simulink model "Sim_Helikopter"  (R2015b)
settings: Solver=ode113  StartTime=0.0  StopTime=50  RelTol=1e-2
PostLoadFcn:
  | , if any(exist('dsrtsu_mdlpostloadfcn', 'file') == [2, 3, 6]), try dsrtsu_mdlpostloadfcn('Execute', bdroot); catch fprintf('Error in PostLoadFcn (dsrtsu_mdlpostloadfcn) for model "%s":\n %s\n', bdroot, lasterr); end, end,
InitFcn:
  | Initialisierung
values from neighbouring files (symbols this model uses):
  initCond = block.DialogPrm(2).Data    [ROFLcopter_modell_S.m]    (also in set_parameter_vollstaendigesModell.m = [0,0,q20,0,0,0,0,0,0,0,0,0]')
  parameters = p    [set_parameter_vollstaendigesModell.m]
  q10e = 0    [Initialisierung.m]
  q1d = 2*pi    (= 6.28318530718)    [Initialisierung.m]
  q20e = 0.319187912478128    (= 0.319187912478)    [Initialisierung.m]
  q2d = 0    [Initialisierung.m]
  sysPar = block.DialogPrm(1).Data    [ROFLcopter_modell_S.m]
  Ta = 1e-3    (= 0.001)    [Initialisierung.m]    (also in Initialisierung_bitte_vervollstaendigen.m)
undefined symbols (not defined in the file or in its folder): F2U, Fout, regPar
settings Model: DSRTSU_INTERNAL_RTI_VER=340  DSRTSU_INTERNAL_RTI_TYPE=rti1103  ExtModeArmWhenConnect=off  Creator=tk  LastModifiedBy=Andreas
settings DataIOCC: SaveFormat=Array  SignalLoggingSaveFormat=ModelDataLogs  SignalLoggingName=sigsOut
settings OptimizationCC: ConditionallyExecuteInputs=off  OptimizeBlockIOStorage=off  BufferReuse=off  GlobalBufferReuse=off  ExpressionFolding=off  ExpressionDepthLimit=2147483647  LocalBlockOutputs=off  InitFltsAndDblsToZero=on
settings DebuggingCC: SaveWithParameterizedLinksMsg=none  UnderspecifiedInitializationDetection=Classic  MergeDetectMultiDrivingBlocksExec=none  SignalResolutionControl=TryResolveAllWithWarning  MultiTaskDSMMsg=warning  MultiTaskCondExecSysMsg=none  FcnCallInpInsideContextMsg=UseLocalSettings  StateNameClashWarn=warning
settings HardwareCC: ProdBitPerPointer=32  ProdLargestAtomicFloat=None  ProdIntDivRoundTo=Undefined  ProdEndianess=Unspecified  ProdWordSize=32  ProdHWDeviceType=32-bit Generic  TargetBitPerLong=64  TargetBitPerPointer=64  TargetLongLongMode=on  TargetIntDivRoundTo=Zero  TargetEndianess=LittleEndian  TargetWordSize=64  TargetHWDeviceType=MATLAB Host  ProdEqTarget=off
settings SFSimCC: SimParseCustomCode=off
settings RTWCC: SystemTargetFile=rtwsfcn.tlc  TemplateMakefile=rtwsfcn_default_tmf  Description=S-function Target  RetainRTWFile=on  RTWCompilerOptimization=on
settings STFCustomTargetCC: ModelReferenceCompliant=off  CompOptLevelCompliant=on  ConcurrentExecutionCompliant=off  MATLABClassNameForMDSCustomization=Simulink.SoftwareTarget.TargetSpecificTriggerConfigurationBase  CPPClassGenCompliant=off  SystemTargetFile=rtwsfcn.tlc
settings ConfigComp: CovModelRefEnable=Off

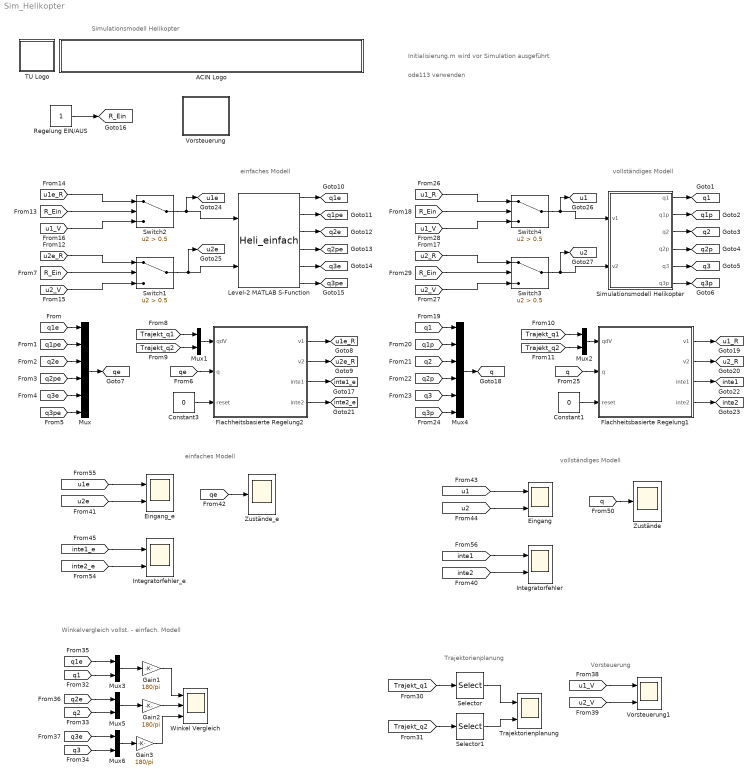
== system Sim_Helikopter ==
  note: ode113 verwenden
  note: Initialisierung.m wird vor Simulation ausgeführt
  note: vollständiges Modell
  note: einfaches Modell
  note: Simulationsmodell Helikopter
  note: Winkelvergleich vollst. - einfach. Modell
  note: Trajektorienplanung
  note: Vorsteuerung
  note: einfaches Modell
  note: vollständiges Modell
  ACIN Logo : Subsystem
      mask init:
      | s = get_param(gcb,'UserData');
      mask Display:
      | image(s.logo,[0 0 439 45]);
      | %axis image
  Constant1 : Constant  Value=0
  Constant3 : Constant  Value=0
  Eingang : Scope  NumInputPorts=2
  Eingang_e : Scope  NumInputPorts=2
  Flachheitsbasierte Regelung1 : MATLAB Function  TreatAsAtomicUnit=on
  Flachheitsbasierte Regelung2 : MATLAB Function  TreatAsAtomicUnit=on
  Gain1 : Gain  Gain=180/pi  SaturateOnIntegerOverflow=on  OutDataTypeStr=Inherit: Same as input  ParamDataTypeStr=Inherit: Same as input
  Gain2 : Gain  Gain=180/pi  SaturateOnIntegerOverflow=on  OutDataTypeStr=Inherit: Same as input  ParamDataTypeStr=Inherit: Same as input
  Gain3 : Gain  Gain=180/pi  SaturateOnIntegerOverflow=on  OutDataTypeStr=Inherit: Same as input  ParamDataTypeStr=Inherit: Same as input
  Integratorfehler : Scope  NumInputPorts=2
  Integratorfehler_e : Scope  NumInputPorts=2
  Level-2 MATLAB S-Function : M-S-Function  FunctionName=Heli_einfach  Parameters=sysPar.xR [sysPar.a1 sysPar.a2 sysPar.a3 sysPar.b1 sysPar.b2 sysPar.b3]
  Mux : Mux  Inputs=6
  Mux{1..3,5..6} (5 alike) : Mux  Inputs=2
  Mux4 : Mux  Inputs=6
  Regelung EIN/AUS : Constant
  Selector : Selector  InputPortWidth=5  IndexOptions=Index vector (dialog)  Indices=1  OutputSizes=1
  Selector1 : Selector  InputPortWidth=5  IndexOptions=Index vector (dialog)  Indices=1  OutputSizes=1
  Simulationsmodell Helikopter : Subsystem
  Switch{1..4} (4 alike) : Switch  Criteria=u2 > Threshold  Threshold=0.5
  TU Logo : Subsystem
      mask init:
      | s = get_param(gcb,'UserData');
      mask Display: image(s.logo,[0 0 45 45]);
  Trajektorienplanung : Scope  NumInputPorts=2
  Vorsteuerung : Subsystem
  Vorsteuerung1 : Scope  NumInputPorts=2
  Winkel Vergleich : Scope  NumInputPorts=3
  "Zustände " : Scope
  Zustände_e : Scope
  tag scope: R_Ein=global, inte1=global, inte1_e=global, inte2=global, inte2_e=global, q1=global, q1e=global, q1p=global, q1pe=global, q2=global, q2e=global, q2p=global, q2pe=global, q3=global, q3e=global, q3p=global, q3pe=global, q=global, qe=global, u1=global, u1_R=global, u1e=global, u1e_R=global, u2=global, u2_R=global, u2e=global, u2e_R=global
  wires:
  Simulationsmodell Helikopter/1(q1) -> [q1]
  Simulationsmodell Helikopter/2(q1p) -> [q1p]
  Simulationsmodell Helikopter/3(q2) -> [q2]
  Simulationsmodell Helikopter/4(q2p) -> [q2p]
  Simulationsmodell Helikopter/5(q3) -> [q3]
  Simulationsmodell Helikopter/6(q3p) -> [q3p]
  Mux/1 -> [qe]
  [q1e] -> Mux/1
  [q1pe] -> Mux/2
  [q2e] -> Mux/3
  [q2pe] -> Mux/4
  [q3e] -> Mux/5
  [q3pe] -> Mux/6
  Level-2 MATLAB S-Function/6 -> [q3pe]
  Level-2 MATLAB S-Function/5 -> [q3e]
  Level-2 MATLAB S-Function/4 -> [q2pe]
  Level-2 MATLAB S-Function/3 -> [q2e]
  Level-2 MATLAB S-Function/2 -> [q1pe]
  Level-2 MATLAB S-Function/1 -> [q1e]
  Mux4/1 -> [q]
  [q1] -> Mux4/1
  [q1p] -> Mux4/2
  [q2] -> Mux4/3
  [q2p] -> Mux4/4
  [q3] -> Mux4/5
  [q3p] -> Mux4/6
  Flachheitsbasierte Regelung1/1(v1) -> [u1_R]
  Flachheitsbasierte Regelung1/2(v2) -> [u2_R]
  Constant1/1 -> Flachheitsbasierte Regelung1/3(reset)
  [q] -> Flachheitsbasierte Regelung1/2(q)
  Flachheitsbasierte Regelung1/3(inte1) -> [inte1]
  Flachheitsbasierte Regelung1/4(inte2) -> [inte2]
  Flachheitsbasierte Regelung2/1(v1) -> [u1e_R]
  Flachheitsbasierte Regelung2/2(v2) -> [u2e_R]
  Constant3/1 -> Flachheitsbasierte Regelung2/3(reset)
  Mux1/1 -> Flachheitsbasierte Regelung2/1(qdV)
  [qe] -> Flachheitsbasierte Regelung2/2(q)
  Flachheitsbasierte Regelung2/3(inte1) -> [inte1_e]
  Flachheitsbasierte Regelung2/4(inte2) -> [inte2_e]
  Switch2/1 -> [u1e], Level-2 MATLAB S-Function/1
  [Trajekt_q1] -> Mux1/1
  [Trajekt_q2] -> Mux1/2
  [Trajekt_q1] -> Mux2/1
  [Trajekt_q2] -> Mux2/2
  Mux2/1 -> Flachheitsbasierte Regelung1/1(qdV)
  [R_Ein] -> Switch2/2
  [u1e_R] -> Switch2/1
  [u1_V] -> Switch2/3
  [R_Ein] -> Switch1/2
  [u2e_R] -> Switch1/1
  [u2_V] -> Switch1/3
  Switch1/1 -> [u2e], Level-2 MATLAB S-Function/2
  Switch4/1 -> [u1], Simulationsmodell Helikopter/1(v1)
  [R_Ein] -> Switch4/2
  [u1_R] -> Switch4/1
  [u1_V] -> Switch4/3
  [R_Ein] -> Switch3/2
  [u2_R] -> Switch3/1
  [u2_V] -> Switch3/3
  Switch3/1 -> [u2], Simulationsmodell Helikopter/2(v2)
  Regelung EIN/AUS/1 -> [R_Ein]
  [q3] -> Mux6/2
  [q2] -> Mux5/2
  [q1] -> Mux3/2
  [q3e] -> Mux6/1
  [q2e] -> Mux5/1
  [q1e] -> Mux3/1
  [u1_V] -> Vorsteuerung1/1
  [u2_V] -> Vorsteuerung1/2
  [u1] -> Eingang/1
  [u2] -> Eingang/2
  Gain1/1 -> Winkel Vergleich/1
  Mux3/1 -> Gain1/1
  Gain2/1 -> Winkel Vergleich/2
  Mux5/1 -> Gain2/1
  Mux6/1 -> Gain3/1
  Gain3/1 -> Winkel Vergleich/3
  [inte1] -> Integratorfehler/1
  [inte2] -> Integratorfehler/2
  [u1e] -> Eingang_e/1
  [u2e] -> Eingang_e/2
  [inte1_e] -> Integratorfehler_e/1
  [inte2_e] -> Integratorfehler_e/2
  [q] -> "Zustände "/1
  [qe] -> Zustände_e/1
  [Trajekt_q1] -> Selector/1
  Selector/1 -> Trajektorienplanung/1
  [Trajekt_q2] -> Selector1/1
  Selector1/1 -> Trajektorienplanung/2

== system Sim_Helikopter/ACIN Logo ==

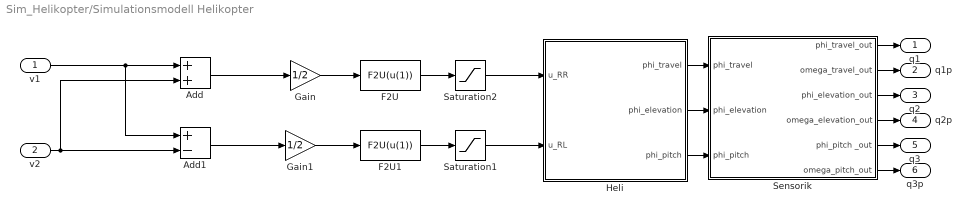
== system Sim_Helikopter/Simulationsmodell Helikopter ==
  v1 : Inport
  v2 : Inport  Port=2
  Add : Sum
  Add1 : Sum  Inputs=+-
  F2U : MATLABFcn  MATLABFcn=F2U(u(1))  OutputDimensions=1  Output1D=off
  F2U1 : MATLABFcn  MATLABFcn=F2U(u(1))  OutputDimensions=1  Output1D=off
  Gain : Gain  Gain=1/2
  Gain1 : Gain  Gain=1/2
  Heli : Subsystem
  Saturation1 : Saturate  UpperLimit=15  LowerLimit=-15
  Saturation2 : Saturate  UpperLimit=15  LowerLimit=-15
  Sensorik : Subsystem
  q1 : Outport
  q1p : Outport  Port=2
  q2 : Outport  Port=3
  q2p : Outport  Port=4
  q3 : Outport  Port=5
  q3p : Outport  Port=6
  wires:
  Saturation1/1 -> Heli/2(u_RL)
  Saturation2/1 -> Heli/1(u_RR)
  Heli/1(phi_travel) -> Sensorik/1(phi_travel)
  Heli/2(phi_elevation) -> Sensorik/2(phi_elevation)
  Heli/3(phi_pitch) -> Sensorik/3(phi_pitch)
  Sensorik/1(phi_travel_out) -> q1/1
  Sensorik/2(omega_travel_out) -> q1p/1
  Sensorik/3(phi_elevation_out) -> q2/1
  Sensorik/4(omega_elevation_out) -> q2p/1
  Sensorik/5(phi_pitch _out) -> q3/1
  Sensorik/6(omega_pitch_out) -> q3p/1
  v1/1 -> Add/1, Add1/1
  v2/1 -> Add/2, Add1/2
  Add/1 -> Gain/1
  Add1/1 -> Gain1/1
  Gain/1 -> F2U/1
  Gain1/1 -> F2U1/1
  F2U/1 -> Saturation2/1
  F2U1/1 -> Saturation1/1

== system Sim_Helikopter/TU Logo ==

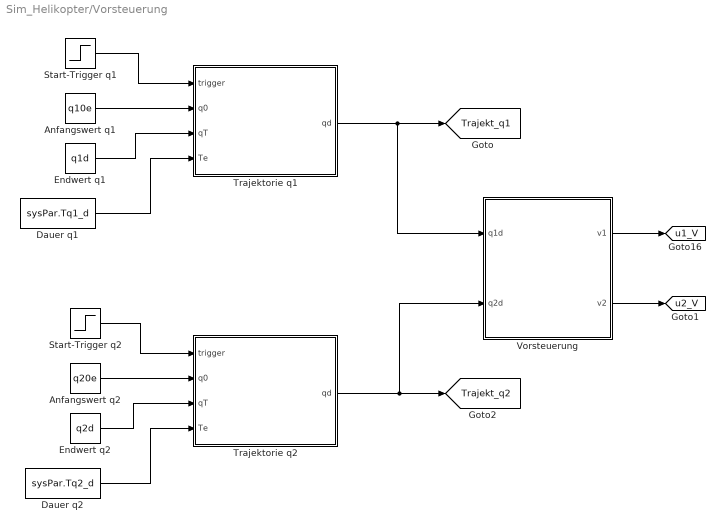
== system Sim_Helikopter/Vorsteuerung ==
  Anfangswert q1 : Constant  Value=q10e
  Anfangswert q2 : Constant  Value=q20e
  Dauer q1 : Constant  Value=sysPar.Tq1_d
  Dauer q2 : Constant  Value=sysPar.Tq2_d
  Endwert q1 : Constant  Value=q1d
  Endwert q2 : Constant  Value=q2d
  Start-Trigger q1 : Step  Time=sysPar.Tq1_s  SampleTime=0
  Start-Trigger q2 : Step  Time=sysPar.Tq2_s  SampleTime=0
  Trajektorie q1 : MATLAB Function  TreatAsAtomicUnit=on
  Trajektorie q2 : MATLAB Function  TreatAsAtomicUnit=on
  "Vorsteuerung " : MATLAB Function  TreatAsAtomicUnit=on
  tag scope: Trajekt_q1=global, Trajekt_q2=global, u1_V=global, u2_V=global
  wires:
  Start-Trigger q1/1 -> Trajektorie q1/1(trigger)
  Anfangswert q1/1 -> Trajektorie q1/2(q0)
  Endwert q1/1 -> Trajektorie q1/3(qT)
  Start-Trigger q2/1 -> Trajektorie q2/1(trigger)
  Anfangswert q2/1 -> Trajektorie q2/2(q0)
  Endwert q2/1 -> Trajektorie q2/3(qT)
  Trajektorie q1/1(qd) -> [Trajekt_q1], "Vorsteuerung "/1(q1d)
  Dauer q2/1 -> Trajektorie q2/4(Te)
  Dauer q1/1 -> Trajektorie q1/4(Te)
  Trajektorie q2/1(qd) -> [Trajekt_q2], "Vorsteuerung "/2(q2d)
  "Vorsteuerung "/2(v2) -> [u2_V]
  "Vorsteuerung "/1(v1) -> [u1_V]

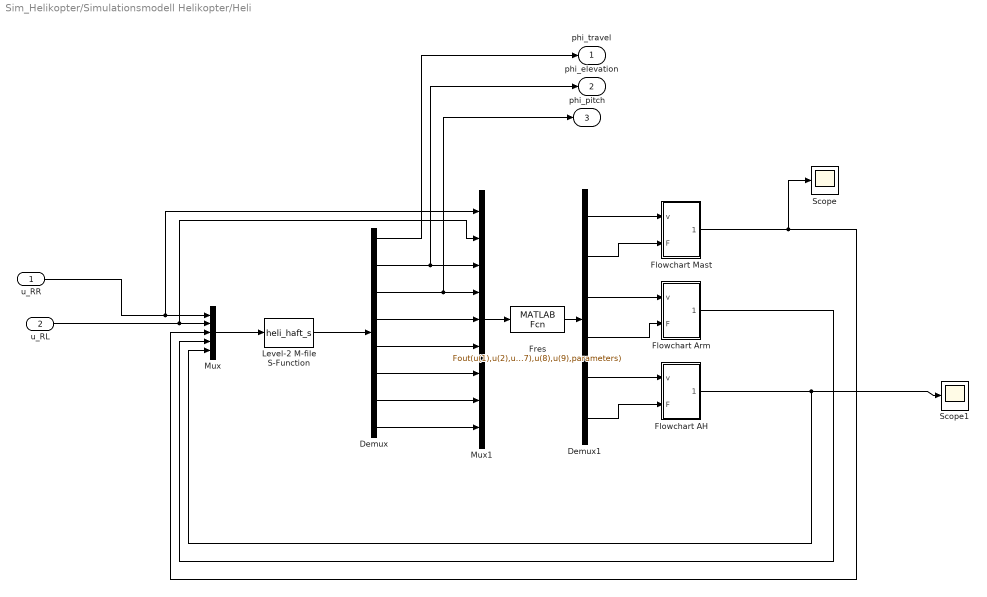
== system Sim_Helikopter/Simulationsmodell Helikopter/Heli ==
  u_RR : Inport
  u_RL : Inport  Port=2
  Demux : Demux  Outputs=8
  Demux1 : Demux  Outputs=6
  Flowchart AH : Subsystem
  Flowchart Arm : Subsystem
  Flowchart Mast : Subsystem
  Fres : MATLABFcn  MATLABFcn=Fout(u(1),u(2),u(3),u(4),u(5),u(6),u(7),u(8),u(9),parameters)  OutputDimensions=6  Output1D=off
  Level-2 M-file S-Function : M-S-Function  FunctionName=heli_haft_s  Parameters=initCond, parameters
  Mux : Mux  Inputs=5
  Mux1 : Mux  Inputs=9
  Scope : Scope
  Scope1 : Scope
  phi_travel : Outport
  phi_elevation : Outport  Port=2
  phi_pitch : Outport  Port=3
  wires:
  Demux/1 -> phi_travel/1
  u_RR/1 -> Mux1/1, Mux/1
  u_RL/1 -> Mux1/2, Mux/2
  Demux1/6 -> Flowchart AH/2(F)
  Demux1/5 -> Flowchart AH/1(v)
  Demux1/4 -> Flowchart Arm/2(F)
  Demux1/3 -> Flowchart Arm/1(v)
  Demux1/2 -> Flowchart Mast/2(F)
  Demux1/1 -> Flowchart Mast/1(v)
  Fres/1 -> Demux1/1
  Mux1/1 -> Fres/1
  Demux/2 -> Mux1/3, phi_elevation/1
  Demux/3 -> Mux1/4, phi_pitch/1
  Demux/4 -> Mux1/5
  Demux/5 -> Mux1/6
  Demux/6 -> Mux1/7
  Demux/7 -> Mux1/8
  Demux/8 -> Mux1/9
  Flowchart Mast/1(Out1) -> Mux/3, Scope/1
  Flowchart Arm/1(Out1) -> Mux/4
  Flowchart AH/1(Out1) -> Scope1/1, Mux/5
  Level-2 M-file S-Function/1 -> Demux/1
  Mux/1 -> Level-2 M-file S-Function/1

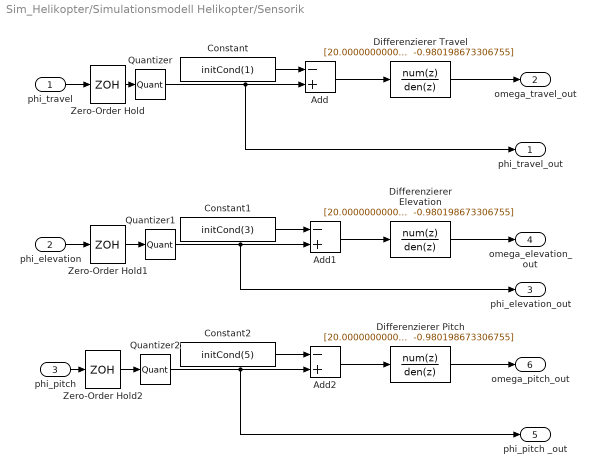
== system Sim_Helikopter/Simulationsmodell Helikopter/Sensorik ==
  phi_travel : Inport
  phi_elevation : Inport  Port=2
  phi_pitch : Inport  Port=3
  Add : Sum  Inputs=-+
  Add1 : Sum  Inputs=-+
  Add2 : Sum  Inputs=-+
  Constant : Constant  Value=initCond(1)
  Constant1 : Constant  Value=initCond(3)
  Constant2 : Constant  Value=initCond(5)
  Differenzierer Elevation : DiscreteTransferFcn  Numerator=[20.000000000000000 -19.999999999999996]  Denominator="[1.000000000000000  -0.980198673306755]"  SampleTime=1e-3
  Differenzierer Pitch : DiscreteTransferFcn  Numerator=[20.000000000000000 -19.999999999999996]  Denominator="[1.000000000000000  -0.980198673306755]"  SampleTime=1e-3
  Differenzierer Travel : DiscreteTransferFcn  Numerator=[20.000000000000000 -19.999999999999996]  Denominator="[1.000000000000000  -0.980198673306755]"  SampleTime=1e-3
  Quantizer : Quantizer  QuantizationInterval=2*pi/2^13
  Quantizer1 : Quantizer  QuantizationInterval=2*pi/4096
  Quantizer2 : Quantizer  QuantizationInterval=2*pi/4096
  Zero-Order Hold : ZeroOrderHold  SampleTime=1e-3
  Zero-Order Hold1 : ZeroOrderHold  SampleTime=1e-3
  Zero-Order Hold2 : ZeroOrderHold  SampleTime=1e-3
  phi_travel_out : Outport
  omega_travel_out : Outport  Port=2
  phi_elevation_out : Outport  Port=3
  omega_elevation_out : Outport  Port=4
  phi_pitch _out : Outport  Port=5
  omega_pitch_out : Outport  Port=6
  wires:
  Zero-Order Hold/1 -> Quantizer/1
  Quantizer/1 -> phi_travel_out/1, Add/2
  Zero-Order Hold1/1 -> Quantizer1/1
  Quantizer1/1 -> phi_elevation_out/1, Add1/2
  Zero-Order Hold2/1 -> Quantizer2/1
  Quantizer2/1 -> phi_pitch _out/1, Add2/2
  Differenzierer Travel/1 -> omega_travel_out/1
  phi_travel/1 -> Zero-Order Hold/1
  Differenzierer Elevation/1 -> omega_elevation_out/1
  phi_elevation/1 -> Zero-Order Hold1/1
  Differenzierer Pitch/1 -> omega_pitch_out/1
  phi_pitch/1 -> Zero-Order Hold2/1
  Add/1 -> Differenzierer Travel/1
  Add1/1 -> Differenzierer Elevation/1
  Add2/1 -> Differenzierer Pitch/1
  Constant/1 -> Add/1
  Constant1/1 -> Add1/1
  Constant2/1 -> Add2/1

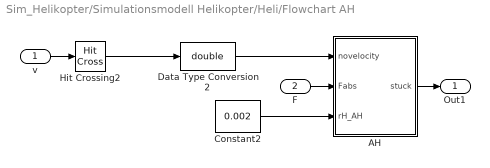
== system Sim_Helikopter/Simulationsmodell Helikopter/Heli/Flowchart AH ==
  v : Inport
  F : Inport  Port=2
  AH : Stateflow chart  TreatAsAtomicUnit=on
  Constant2 : Constant  Value=0.002
  Data Type Conversion2 : DataTypeConversion  OutDataTypeStr=double  SaturateOnIntegerOverflow=on  RndMeth=Zero
  Hit Crossing2 : HitCross  ZeroCross=off
  Out1 : Outport
  wires:
  AH/1(stuck) -> Out1/1
  F/1 -> AH/2(Fabs)
  v/1 -> Hit Crossing2/1
  Constant2/1 -> AH/3(rH_AH)
  Data Type Conversion2/1 -> AH/1(novelocity)
  Hit Crossing2/1 -> Data Type Conversion2/1

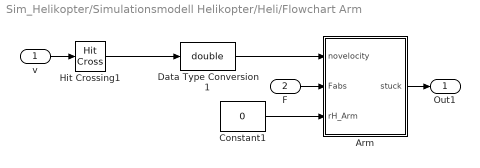
== system Sim_Helikopter/Simulationsmodell Helikopter/Heli/Flowchart Arm ==
  v : Inport
  F : Inport  Port=2
  Arm : Stateflow chart  TreatAsAtomicUnit=on
  Constant1 : Constant  Value=0
  Data Type Conversion1 : DataTypeConversion  OutDataTypeStr=double  SaturateOnIntegerOverflow=on  RndMeth=Zero
  Hit Crossing1 : HitCross  ZeroCross=off
  Out1 : Outport
  wires:
  Arm/1(stuck) -> Out1/1
  F/1 -> Arm/2(Fabs)
  v/1 -> Hit Crossing1/1
  Hit Crossing1/1 -> Data Type Conversion1/1
  Data Type Conversion1/1 -> Arm/1(novelocity)
  Constant1/1 -> Arm/3(rH_Arm)

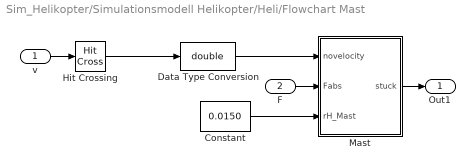
== system Sim_Helikopter/Simulationsmodell Helikopter/Heli/Flowchart Mast ==
  v : Inport
  F : Inport  Port=2
  Constant : Constant  Value=0.0150
  Data Type Conversion : DataTypeConversion  OutDataTypeStr=double  SaturateOnIntegerOverflow=on  RndMeth=Zero
  Hit Crossing : HitCross  ZeroCross=off
  Mast : Stateflow chart  TreatAsAtomicUnit=on
  Out1 : Outport
  wires:
  Mast/1(stuck) -> Out1/1
  F/1 -> Mast/2(Fabs)
  v/1 -> Hit Crossing/1
  Constant/1 -> Mast/3(rH_Mast)
  Data Type Conversion/1 -> Mast/1(novelocity)
  Hit Crossing/1 -> Data Type Conversion/1

== matlab function Sim_Helikopter/Vorsteuerung/Trajektorie q1 ==
  settings: updateMethod=DISCRETE  sampleTime=Ta
  data: trigger input; qd output; q0 input; qT input; Te input; sysPar parameter
function qd  = feedfw_q1(trigger,q0,qT,Te,sysPar)


beta5 = sysPar.beta5;
beta6 = sysPar.beta6;
beta7 = sysPar.beta7;
beta8 = sysPar.beta8;
beta9 = sysPar.beta9;


persistent t;

Ta=sysPar.Ta;
T=Te;
if isempty(t)
    t=0;
end
if(trigger)
    q=q0 + (qT-q0) * (beta5*(t/T)^5+beta6*(t/T)^6+beta7*(t/T)^7+beta8*(t/T)^8+beta9*(t/T)^9);
    qp=(qT - q0) * (5 * beta5 * t ^ 4 / T ^ 5 + 6 * beta6 * t ^ 5 / T ^ 6 + 7 * beta7 * t ^ 6 / T ^ 7 + 8 * beta8 * t ^ 7 / T ^ 8 + 9 * beta9 * t ^ 8 / T ^ 9);
    qpp=(qT - q0) * (20 * beta5 * t ^ 3 / T ^ 5 + 30 * beta6 * t ^ 4 / T ^ 6 + 42 * beta7 * t ^ 5 / T ^ 7 + 56 * beta8 * t ^ 6 / T ^ 8 + 72 * beta9 * t ^ 7 / T ^ 9);
    qppp=(qT - q0) * (60 * beta5 * t ^ 2 / T ^ 5 + 120 * beta6 * t ^ 3 / T ^ 6 + 210 * beta7 * t ^ 4 / T ^ 7 + 336 * beta8 * t ^ 5 / T ^ 8 + 504 * beta9 * t ^ 6 / T ^ 9); 
    qpppp=(qT - q0) * (120 * beta5 * t / T ^ 5 + 360 * beta6 * t ^ 2 / T ^ 6 + 840 * beta7 * t ^ 3 / T ^ 7 + 1680 * beta8 * t ^ 4 / T ^ 8 + 3024 * beta9 * t ^ 5 / T ^ 9);

    if t<T
        t=t+Ta;
        qd=[q;qp;qpp;qppp;qpppp];
    else
        qd=[qT;0;0;0;0];  
    end
    
else
    qd=[q0;0;0;0;0];
end

== matlab function Sim_Helikopter/Vorsteuerung/Trajektorie q2 ==
  settings: updateMethod=DISCRETE  sampleTime=Ta
  data: trigger input; qd output; q0 input; qT input; Te input; sysPar parameter
function qd  = feedfw_q2(trigger,q0,qT,Te,sysPar)

beta5 = sysPar.beta5;
beta6 = sysPar.beta6;
beta7 = sysPar.beta7;
beta8 = sysPar.beta8;
beta9 = sysPar.beta9;


persistent t;

Ta=sysPar.Ta;
T=Te;
if isempty(t)
    t=0;
end
if(trigger)
    q=q0 + (qT-q0) * (beta5*(t/T)^5+beta6*(t/T)^6+beta7*(t/T)^7+beta8*(t/T)^8+beta9*(t/T)^9);
    qp=(qT - q0) * (5 * beta5 * t ^ 4 / T ^ 5 + 6 * beta6 * t ^ 5 / T ^ 6 + 7 * beta7 * t ^ 6 / T ^ 7 + 8 * beta8 * t ^ 7 / T ^ 8 + 9 * beta9 * t ^ 8 / T ^ 9);
    qpp=(qT - q0) * (20 * beta5 * t ^ 3 / T ^ 5 + 30 * beta6 * t ^ 4 / T ^ 6 + 42 * beta7 * t ^ 5 / T ^ 7 + 56 * beta8 * t ^ 6 / T ^ 8 + 72 * beta9 * t ^ 7 / T ^ 9);
    qppp=(qT - q0) * (60 * beta5 * t ^ 2 / T ^ 5 + 120 * beta6 * t ^ 3 / T ^ 6 + 210 * beta7 * t ^ 4 / T ^ 7 + 336 * beta8 * t ^ 5 / T ^ 8 + 504 * beta9 * t ^ 6 / T ^ 9); 
    qpppp=(qT - q0) * (120 * beta5 * t / T ^ 5 + 360 * beta6 * t ^ 2 / T ^ 6 + 840 * beta7 * t ^ 3 / T ^ 7 + 1680 * beta8 * t ^ 4 / T ^ 8 + 3024 * beta9 * t ^ 5 / T ^ 9);
     
    if t<=T
        t=t+Ta;
        qd=[q;qp;qpp;qppp;qpppp];
    else
        qd=[qT;0;0;0;0];  
    end
    
else
    qd=[q0;0;0;0;0];
end

== matlab function Sim_Helikopter/Vorsteuerung/Vorsteuerung  ==
  settings: updateMethod=DISCRETE  sampleTime=Ta
  data: q1d input; v1 output; q2d input; sysPar parameter; v2 output
function [v1,v2] = fcn(q1d,q2d,sysPar)


q1pp=q1d(3);
q1ppp=q1d(4);
q1pppp=q1d(5);

a1=sysPar.a1;
a2=sysPar.a2;
a3=sysPar.a3;
b1=sysPar.b1;
b2=sysPar.b2;
b3=sysPar.b3;

q2=q2d(1);
q2p=q2d(2);
q2pp=q2d(3);
q2ppp=q2d(4);
q2pppp=q2d(5);

v1 = -0.1e1 / b2 * (a1 * sin(q2) + a2 * cos(q2) - q2pp) * sqrt(b2 ^ 2 * q1pp ^ 2 / b1 ^ 2 / cos(q2) ^ 2 / (a1 * sin(q2) + a2 * cos(q2) - q2pp) ^ 2 + 0.1e1);
v2 = -(-a3 * b2 * q1pp / b1 / (a1 * sin(q2) + a2 * cos(q2) - q2pp) * (b2 ^ 2 * q1pp ^ 2 / b1 ^ 2 / cos(q2) ^ 2 / (a1 * sin(q2) + a2 * cos(q2) - q2pp) ^ 2 + 0.1e1) ^ (-0.1e1 / 0.2e1) - b2 * ((-a1 * sin(q2) - a2 * cos(q2) + q2pp) * cos(q2) * (b2 ^ 2 * q1pp ^ 2 + b1 ^ 2 * cos(q2) ^ 2 * (-a1 * sin(q2) - a2 * cos(q2) + q2pp) ^ 2) * q1pppp - q1pp * cos(q2) * (b2 ^ 2 * q1pp ^ 2 + b1 ^ 2 * cos(q2) ^ 2 * (-a1 * sin(q2) - a2 * cos(q2) + q2pp) ^ 2) * q2pppp - 0.2e1 * q1pp * b2 ^ 2 * cos(q2) * (-a1 * sin(q2) - a2 * cos(q2) + q2pp) * q1ppp ^ 2 - 0.2e1 * (b2 * q1pp - b1 * cos(q2) * (-a1 * sin(q2) - a2 * cos(q2) + q2pp)) * (-cos(q2) * q2ppp + q2p * (a1 * cos(q2) ^ 2 - a1 * sin(q2) ^ 2 - 0.2e1 * a2 * sin(q2) * cos(q2) + q2pp * sin(q2))) * (b2 * q1pp + b1 * cos(q2) * (-a1 * sin(q2) - a2 * cos(q2) + q2pp)) * q1ppp + q1pp * (0.2e1 * b1 ^ 2 * cos(q2) ^ 3 * (-a1 * sin(q2) - a2 * cos(q2) + q2pp) * q2ppp ^ 2 + 0.2e1 * (q1pp ^ 2 * b2 ^ 2 * sin(q2) - b1 ^ 2 * cos(q2) ^ 2 * (0.2e1 * a1 * cos(q2) ^ 2 - a1 * sin(q2) ^ 2 - 0.3e1 * a2 * sin(q2) * cos(q2) + q2pp * sin(q2)) * (-a1 * sin(q2) - a2 * cos(q2) + q2pp)) * q2p * q2ppp + (q2pp ^ 2 * sin(q2) + (q2p ^ 2 * cos(q2) + a1 * cos(q2) ^ 2 - a1 * sin(q2) ^ 2 - 0.2e1 * a2 * sin(q2) * cos(q2)) * q2pp - 0.4e1 * (a1 * cos(q2) * sin(q2) + a2 * cos(q2) ^ 2 / 0.2e1 - a2 * sin(q2) ^ 2 / 0.2e1) * q2p ^ 2) * b2 ^ 2 * q1pp ^ 2 + (q2pp ^ 3 * cos(q2) * sin(q2) + ((cos(q2) ^ 2 + 0.2e1 * sin(q2) ^ 2) * q2p ^ 2 + cos(q2) * (a1 * cos(q2) ^ 2 - 0.2e1 * a1 * sin(q2) ^ 2 - 0.3e1 * a2 * sin(q2) * cos(q2))) * q2pp ^ 2 + ((-a1 * cos(q2) ^ 2 * sin(q2) - 0.4e1 * a1 * sin(q2) ^ 3 - 0.3e1 * a2 * cos(q2) ^ 3 - 0.6e1 * a2 * cos(q2) * sin(q2) ^ 2) * q2p ^ 2 - cos(q2) * (a1 * cos(q2) ^ 2 - a1 * sin(q2) ^ 2 - 0.2e1 * a2 * sin(q2) * cos(q2)) * (a1 * sin(q2) + a2 * cos(q2))) * q2pp + 0.2e1 * ((a1 ^ 2 + a2 ^ 2) * cos(q2) ^ 4 - a1 * a2 * cos(q2) ^ 3 * sin(q2) + 0.3e1 * a2 ^ 2 * cos(q2) ^ 2 * sin(q2) ^ 2 + 0.3e1 * a1 * a2 * cos(q2) * sin(q2) ^ 3 + a1 ^ 2 * sin(q2) ^ 4) * q2p ^ 2) * (-a1 * sin(q2) - a2 * cos(q2) + q2pp) * cos(q2) * b1 ^ 2)) * b1 / (b2 ^ 2 * q1pp ^ 2 + b1 ^ 2 * cos(q2) ^ 2 * (-a1 * sin(q2) - a2 * cos(q2) + q2pp) ^ 2) ^ 2) / b3;

== matlab function Sim_Helikopter/Flachheitsbasierte Regelung2 ==
  settings: updateMethod=DISCRETE  sampleTime=Ta
  data: qdV input; q input; sysPar parameter; regPar parameter; reset input; v1 output; v2 output; Ta parameter; inte1 output; inte2 output
function [v1,v2,inte1,inte2] = FLATreg(qdV,q,sysPar,regPar,reset,Ta)
%
% Ta ....... Abtastzeit
% sysPar ... Systemparameter
% regPar ... Reglerparameter
% q ........ Messgrößen
% qdV ...... Sollgrößen aus Trajektorienvorgabe für q1 und q2
% reset .... Reset für dSpace
%
% Persistent Variablen für Integration des Fehlers 
persistent e1I
if isempty(e1I) e1I = double(0); end
persistent e2I
if isempty(e2I) e2I = double(0); end

% Reset der Integratoren für die Fehler
if reset
    e1I=0.0;
    e2I=0.0;
end

% Messgrößen 
q1 = q(1);
q1p= q(2);
q2 = q(3);
q2p= q(4);
q3 = q(5);
q3p= q(6);

% Systemparameter
a1 = sysPar.a1;
a2 = sysPar.a2;
a3 = sysPar.a3;
b1 = sysPar.b1;
b2 = sysPar.b2;
b3 = sysPar.b3;

% Auslesen der Reglerparameter
k13 = regPar.k13;
k12 = regPar.k12;
k11 = regPar.k11;
k10 = regPar.k10;
k1I = regPar.k1I;
k21 = regPar.k21;
k20 = regPar.k20;
k2I = regPar.k2I;

% Sollgrößen mit zeitlichen Ableitungen
q1d     = qdV(1);
q1pd    = qdV(2);
q1ppd   = qdV(3);
q1pppd  = qdV(4);
q1ppppd = qdV(5);

q2d     = qdV(6);
q2pd    = qdV(7);
q2ppd   = qdV(8);
q2pppd  = qdV(9);
q2ppppd = qdV(10);

y1d = q1d;
y1dp = q1pd;
y1dpp = q1ppd;
y1dppp = q1pppd;
y1dpppp = q1ppppd;
y2d = q2d;
y2dp = q2pd;
y2dpp = q2ppd;
y2dppp = q2pppd;
y2dpppp = q2ppppd;

% Integration der Fehler: Hier bitte Integrator (Euler-Vorwärts) für Fehler einfügen!
e1I = e1I + Ta*(q1-q1d);
e2I = e2I + Ta*(q2-q2d);

e2 = q2-q2d;
e2p = q2p-q2pd;

% Ableitungen der Ausgänge
q1pp = 0.1e1 / b2 / cos(q3) * (-a1 * sin(q2) - a2 * cos(q2) - k20 * e2 - k2I * e2I - k21 * e2p + y2dpp) * b1 * cos(q2) * sin(q3);
q2pp = -k20 * e2 - k2I * e2I - k21 * e2p + y2dpp;
e2pp = q2pp-q2ppd;
q1ppp = 0.1e1 / b2 / cos(q3) ^ 2 * (-a1 * sin(q2) - a2 * cos(q2) - k20 * e2 - k2I * e2I - k21 * e2p + y2dpp) * b1 * cos(q2) * sin(q3) ^ 2 * q3p + 0.1e1 / b2 / cos(q3) * (-a1 * q2p * cos(q2) + a2 * q2p * sin(q2) - k2I * e2 - k20 * e2p - k21 * e2pp + y2dppp) * b1 * cos(q2) * sin(q3) - 0.1e1 / b2 / cos(q3) * (-a1 * sin(q2) - a2 * cos(q2) - k20 * e2 - k2I * e2I - k21 * e2p + y2dpp) * b1 * q2p * sin(q2) * sin(q3) + 0.1e1 / b2 * (-a1 * sin(q2) - a2 * cos(q2) - k20 * e2 - k2I * e2I - k21 * e2p + y2dpp) * b1 * cos(q2) * q3p;


q2ppp = -k2I * e2 - k20 * e2p - k21 * e2pp + y2dppp;

% Fehlerterme
e1 = q1-q1d;
e1p = q1p-q1pd;
e1pp = q1pp-q1ppd;
e1ppp = q1ppp-q1pppd;
e2ppp = q2ppp-q2pppd;

% Hier bitte Regelgesetz einfügen!
v1 = 0.1e1 / b2 / cos(q3) * (-a1 * sin(q2) - a2 * cos(q2) - k20 * e2 - k2I * e2I - k21 * e2p + y2dpp);
v2 = ((-cos(q2) ^ 2 * a3 * b1 * (a1 * sin(q2) + a2 * cos(q2) + k20 * e2 + k2I * e2I + k21 * e2p - y2dpp) * sin(q3) - 0.2e1 * a1 * q2p * q3p * cos(q2) ^ 2 * b1 + 0.4e1 * q3p * (a2 * q2p * sin(q2) - k2I * e2 / 0.2e1 - k20 * e2p / 0.2e1 - k21 * e2pp / 0.2e1 + y2dppp / 0.2e1) * b1 * cos(q2) + 0.2e1 * a1 * q2p * q3p * sin(q2) ^ 2 * b1 - 0.2e1 * (-k20 * e2 - k2I * e2I - k21 * e2p + y2dpp) * q2p * q3p * sin(q2) * b1 - b2 * (-k10 * e1 - k1I * e1I - k11 * e1p - k12 * e1pp - k13 * e1ppp + y1dpppp)) * cos(q3) ^ 3 - b1 * sin(q3) * ((-0.2e1 * a2 * q2p ^ 2 + 0.2e1 * a2 * q3p ^ 2 + a1 * (-k20 * e2 - k2I * e2I - k21 * e2p + y2dpp)) * cos(q2) ^ 2 + ((-0.4e1 * a1 * q2p ^ 2 + 0.2e1 * a1 * q3p ^ 2 - 0.2e1 * a2 * (-k20 * e2 - k2I * e2I - k21 * e2p + y2dpp)) * sin(q2) + (-k20 * e2 - k2I * e2I - k21 * e2p + y2dpp) * q2p ^ 2 - 0.2e1 * (-k20 * e2 - k2I * e2I - k21 * e2p + y2dpp) * q3p ^ 2 + k20 * e2p + k2I * e2p + k21 * e2ppp - y2dpppp) * cos(q2) - ((-0.2e1 * a2 * q2p ^ 2 + a1 * (-k20 * e2 - k2I * e2I - k21 * e2p + y2dpp)) * sin(q2) - (-k20 * e2 - k2I * e2I - k21 * e2p + y2dpp) ^ 2 - 0.2e1 * (-k2I * e2 - k20 * e2p - k21 * e2pp + y2dppp) * q2p) * sin(q2)) * cos(q3) ^ 2 - 0.2e1 * b1 * (cos(q2) ^ 2 * a3 * (a1 * sin(q2) + a2 * cos(q2) + k20 * e2 + k2I * e2I + k21 * e2p - y2dpp) * sin(q3) / 0.2e1 + q3p * (a1 * q2p * cos(q2) ^ 2 + (-0.2e1 * a2 * q2p * sin(q2) + k2I * e2 + k20 * e2p + k21 * e2pp - y2dppp) * cos(q2) - q2p * sin(q2) * (a1 * sin(q2) + k20 * e2 + k2I * e2I + k21 * e2p - y2dpp))) * sin(q3) ^ 2 * cos(q3) - 0.2e1 * q3p ^ 2 * cos(q2) * sin(q3) ^ 3 * b1 * (a1 * sin(q2) + a2 * cos(q2) + k20 * e2 + k2I * e2I + k21 * e2p - y2dpp)) / cos(q3) / cos(q2) / b1 / b3 / (sin(q3) ^ 2 + cos(q3) ^ 2) / (a1 * sin(q2) + a2 * cos(q2) + k20 * e2 + k2I * e2I + k21 * e2p - y2dpp);


% Ausgabe der Werte der Fehlerintegratoren
inte1 = e1I;
inte2 = e2I;

end

== stateflow chart Sim_Helikopter/Simulationsmodell Helikopter/Heli/Flowchart AH/AH ==
  state stuck/
    entry: stuck=1;
  state sliding/
    entry: stuck=0;
  (default) -> stuck
  sliding -> stuck : [novelocity & fabs(Fabs)<rH_AH]
  stuck -> sliding : [fabs(Fabs)>rH_AH]
  data: novelocity input boolean; Fabs input double; stuck output double; rH_AH input double

== stateflow chart Sim_Helikopter/Simulationsmodell Helikopter/Heli/Flowchart Arm/Arm ==
  state stuck/
    entry: stuck=1;
  state sliding/
    entry: stuck=0;
  (default) -> stuck
  sliding -> stuck : [novelocity & fabs(Fabs)<rH_Arm]
  stuck -> sliding : [fabs(Fabs)>rH_Arm]
  data: novelocity input boolean; Fabs input double; stuck output double; rH_Arm input double

== stateflow chart Sim_Helikopter/Simulationsmodell Helikopter/Heli/Flowchart Mast/Mast ==
  state stuck/
    entry: stuck=1;
  state sliding/
    entry: stuck=0;
  sliding -> stuck : [novelocity & fabs(Fabs)<rH_Mast]
  stuck -> sliding : [fabs(Fabs)>rH_Mast]
  (default) -> sliding
  data: novelocity input boolean; Fabs input double; stuck output double; rH_Mast input double

== matlab function Sim_Helikopter/Flachheitsbasierte Regelung1 ==
  settings: updateMethod=DISCRETE  sampleTime=Ta
  data: qdV input; q input; sysPar parameter; regPar parameter; reset input; v1 output; v2 output; Ta parameter; inte1 output; inte2 output
function [v1,v2,inte1,inte2] = FLATreg(qdV,q,sysPar,regPar,reset,Ta)
%
% Ta ....... Abtastzeit
% sysPar ... Systemparameter
% regPar ... Reglerparameter
% q ........ Messgrößen
% qdV ...... Sollgrößen aus Trajektorienvorgabe für q1 und q2
% reset .... Reset für dSpace
%
% Persistent Variablen für Integration des Fehlers 
persistent e1I
if isempty(e1I) e1I = double(0); end
persistent e2I
if isempty(e2I) e2I = double(0); end

% Reset der Integratoren für die Fehler
if reset
    e1I=0.0;
    e2I=0.0;
end

% Messgrößen 
q1 = q(1);
q1p= q(2);
q2 = q(3);
q2p= q(4);
q3 = q(5);
q3p= q(6);

% Systemparameter
a1 = sysPar.a1;
a2 = sysPar.a2;
a3 = sysPar.a3;
b1 = sysPar.b1;
b2 = sysPar.b2;
b3 = sysPar.b3;

% Auslesen der Reglerparameter
k13 = regPar.k13;
k12 = regPar.k12;
k11 = regPar.k11;
k10 = regPar.k10;
k1I = regPar.k1I;
k21 = regPar.k21;
k20 = regPar.k20;
k2I = regPar.k2I;

% Sollgrößen mit zeitlichen Ableitungen
q1d     = qdV(1);
q1pd    = qdV(2);
q1ppd   = qdV(3);
q1pppd  = qdV(4);
q1ppppd = qdV(5);

q2d     = qdV(6);
q2pd    = qdV(7);
q2ppd   = qdV(8);
q2pppd  = qdV(9);
q2ppppd = qdV(10);

y1d = q1d;
y1dp = q1pd;
y1dpp = q1ppd;
y1dppp = q1pppd;
y1dpppp = q1ppppd;
y2d = q2d;
y2dp = q2pd;
y2dpp = q2ppd;
y2dppp = q2pppd;
y2dpppp = q2ppppd;

% Integration der Fehler: Hier bitte Integrator (Euler-Vorwärts) für Fehler einfügen!
e1I = e1I + Ta*(q1-q1d);
e2I = e2I + Ta*(q2-q2d);

e2 = q2-q2d;
e2p = q2p-q2pd;

% Ableitungen der Ausgänge
q1pp = 0.1e1 / b2 / cos(q3) * (-a1 * sin(q2) - a2 * cos(q2) - k20 * e2 - k2I * e2I - k21 * e2p + y2dpp) * b1 * cos(q2) * sin(q3);
q2pp = -k20 * e2 - k2I * e2I - k21 * e2p + y2dpp;
e2pp = q2pp-q2ppd;
q1ppp = 0.1e1 / b2 / cos(q3) ^ 2 * (-a1 * sin(q2) - a2 * cos(q2) - k20 * e2 - k2I * e2I - k21 * e2p + y2dpp) * b1 * cos(q2) * sin(q3) ^ 2 * q3p + 0.1e1 / b2 / cos(q3) * (-a1 * q2p * cos(q2) + a2 * q2p * sin(q2) - k2I * e2 - k20 * e2p - k21 * e2pp + y2dppp) * b1 * cos(q2) * sin(q3) - 0.1e1 / b2 / cos(q3) * (-a1 * sin(q2) - a2 * cos(q2) - k20 * e2 - k2I * e2I - k21 * e2p + y2dpp) * b1 * q2p * sin(q2) * sin(q3) + 0.1e1 / b2 * (-a1 * sin(q2) - a2 * cos(q2) - k20 * e2 - k2I * e2I - k21 * e2p + y2dpp) * b1 * cos(q2) * q3p;


q2ppp = -k2I * e2 - k20 * e2p - k21 * e2pp + y2dppp;

% Fehlerterme
e1 = q1-q1d;
e1p = q1p-q1pd;
e1pp = q1pp-q1ppd;
e1ppp = q1ppp-q1pppd;
e2ppp = q2ppp-q2pppd;

% Hier bitte Regelgesetz einfügen!
v1 = 0.1e1 / b2 / cos(q3) * (-a1 * sin(q2) - a2 * cos(q2) - k20 * e2 - k2I * e2I - k21 * e2p + y2dpp);
v2 = ((-cos(q2) ^ 2 * a3 * b1 * (a1 * sin(q2) + a2 * cos(q2) + k20 * e2 + k2I * e2I + k21 * e2p - y2dpp) * sin(q3) - 0.2e1 * a1 * q2p * q3p * cos(q2) ^ 2 * b1 + 0.4e1 * q3p * (a2 * q2p * sin(q2) - k2I * e2 / 0.2e1 - k20 * e2p / 0.2e1 - k21 * e2pp / 0.2e1 + y2dppp / 0.2e1) * b1 * cos(q2) + 0.2e1 * a1 * q2p * q3p * sin(q2) ^ 2 * b1 - 0.2e1 * (-k20 * e2 - k2I * e2I - k21 * e2p + y2dpp) * q2p * q3p * sin(q2) * b1 - b2 * (-k10 * e1 - k1I * e1I - k11 * e1p - k12 * e1pp - k13 * e1ppp + y1dpppp)) * cos(q3) ^ 3 - b1 * sin(q3) * ((-0.2e1 * a2 * q2p ^ 2 + 0.2e1 * a2 * q3p ^ 2 + a1 * (-k20 * e2 - k2I * e2I - k21 * e2p + y2dpp)) * cos(q2) ^ 2 + ((-0.4e1 * a1 * q2p ^ 2 + 0.2e1 * a1 * q3p ^ 2 - 0.2e1 * a2 * (-k20 * e2 - k2I * e2I - k21 * e2p + y2dpp)) * sin(q2) + (-k20 * e2 - k2I * e2I - k21 * e2p + y2dpp) * q2p ^ 2 - 0.2e1 * (-k20 * e2 - k2I * e2I - k21 * e2p + y2dpp) * q3p ^ 2 + k20 * e2p + k2I * e2p + k21 * e2ppp - y2dpppp) * cos(q2) - ((-0.2e1 * a2 * q2p ^ 2 + a1 * (-k20 * e2 - k2I * e2I - k21 * e2p + y2dpp)) * sin(q2) - (-k20 * e2 - k2I * e2I - k21 * e2p + y2dpp) ^ 2 - 0.2e1 * (-k2I * e2 - k20 * e2p - k21 * e2pp + y2dppp) * q2p) * sin(q2)) * cos(q3) ^ 2 - 0.2e1 * b1 * (cos(q2) ^ 2 * a3 * (a1 * sin(q2) + a2 * cos(q2) + k20 * e2 + k2I * e2I + k21 * e2p - y2dpp) * sin(q3) / 0.2e1 + q3p * (a1 * q2p * cos(q2) ^ 2 + (-0.2e1 * a2 * q2p * sin(q2) + k2I * e2 + k20 * e2p + k21 * e2pp - y2dppp) * cos(q2) - q2p * sin(q2) * (a1 * sin(q2) + k20 * e2 + k2I * e2I + k21 * e2p - y2dpp))) * sin(q3) ^ 2 * cos(q3) - 0.2e1 * q3p ^ 2 * cos(q2) * sin(q3) ^ 3 * b1 * (a1 * sin(q2) + a2 * cos(q2) + k20 * e2 + k2I * e2I + k21 * e2p - y2dpp)) / cos(q3) / cos(q2) / b1 / b3 / (sin(q3) ^ 2 + cos(q3) ^ 2) / (a1 * sin(q2) + a2 * cos(q2) + k20 * e2 + k2I * e2I + k21 * e2p - y2dpp);


% Ausgabe der Werte der Fehlerintegratoren
inte1 = e1I;
inte2 = e2I;

end
